simulink model "mpc_bumpless"  (Simulink 7.2)
settings: Solver=ode3  SolverMode=SingleTasking  StartTime=0.0  StopTime=Tstop  RelTol=1e-3
values from neighbouring files (symbols this model uses):
  den = [1 3 2 0.5]    [mpcbumpless.m]
  num = [1 1]    [mpcbumpless.m]
libraries: mpclib x1
settings Model: Creator=jowen  LastModifiedBy=rchen  ExtModeTrigMode=oneshot  ExtModeArmWhenConnect=off
settings SolverCC: ZeroCrossAlgorithm=Non-adaptive
settings DataIOCC: LimitDataPoints=off  SignalLoggingName=sigsOut
settings OptimizationCC: BooleanDataType=off  InlineInvariantSignals=on  InitFltsAndDblsToZero=on  EfficientMapNaN2IntZero=off
settings DebuggingCC: SaveWithParameterizedLinksMsg=none  CheckExecutionContextPreStartOutputMsg=on  CheckExecutionContextRuntimeOutputMsg=on  SignalResolutionControl=TryResolveAllWithWarning  SolverPrmCheckMsg=none  MultiTaskDSMMsg=warning  MultiTaskCondExecSysMsg=none  IntegerOverflowMsg=none  StrictBusMsg=None
settings HardwareCC: TargetEndianess=LittleEndian  TargetHWDeviceType=MATLAB Host  ProdEqTarget=off
settings RTWCC: IncludeERTFirstTime=on
settings GRTTargetCC: TargetFcnLib=ansi_tfl_tmw.mat

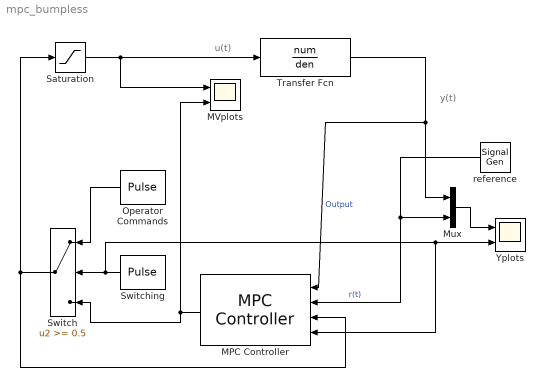
== system mpc_bumpless ==
  note: u(t)
  note: y(t)
  MPC Controller : mpclib/MPC Controller  Orientation=left  SystemSampleTime=-1  mpcobj=MPC1  n_mv=0  x0=[]  ref_from_ws=off  ref_signal_name=[]  ref_preview=on  md_from_ws=off  md_signal_name=[]  md_preview=on  from_project=off  md_inport=off  mv_inport=on  lims_inport=off  switch_inport=on  enable_value=0  project_file=MPCtask.mat  is_multiple=0
  MVplots : Scope  NumInputPorts=2
      settings: TimeRange=250  YMin=-0.6000000000000001~-0.4  YMax=0.3999999999999999~0.4  SaveName=ScopeData2  DataFormat=Structure
  Mux : Mux  Inputs=2
  Operator Commands : DiscretePulseGenerator  Orientation=left  PulseType=Time based  Amplitude=-0.5  Period=180  PulseWidth=50  PhaseDelay=10
  Saturation : Saturate  UpperLimit=1  LowerLimit=-1
  Switch : Switch  Orientation=left  Threshold=0.5
  Switching : DiscretePulseGenerator  Orientation=left  PulseType=Time based  Period=180  PulseWidth=50  PhaseDelay=90
  Transfer Fcn : TransferFcn  Numerator=num  Denominator=den
  Yplots : Scope  NumInputPorts=2
      settings: TimeRange=250  YMin=-1.1~-0.1  YMax=0.6~1.1  SaveName=ScopeData3
  reference : SignalGenerator  Orientation=left  WaveForm=square  Amplitude=0.5  Frequency=.0045
  wires:
  reference/1 -> Mux/2, MPC Controller/2  "r(t)"
  Transfer Fcn/1 -> MPC Controller/1, Mux/1  "Output"
  Switch/1 -> Saturation/1, MPC Controller/3
  Switching/1 -> Switch/2, Yplots/2, MPC Controller/4
  Saturation/1 -> Transfer Fcn/1, MVplots/1
  Mux/1 -> Yplots/1
  MPC Controller/1 -> Switch/3, MVplots/2
  Operator Commands/1 -> Switch/1
